simulink model "simulation_from_file"  (Simulink 7.8)
settings: Solver=ode45  StartTime=0.0  StopTime=5.  RelTol=1e-3
settings Model: Creator=roberto  LastModifiedBy=roberto

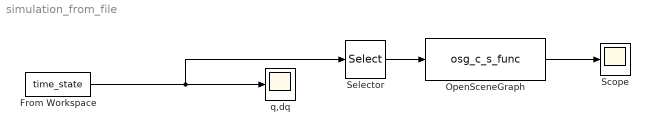
== system simulation_from_file ==
  From Workspace : FromWorkspace  VariableName=time_state  SampleTime=0
  OpenSceneGraph : S-Function  FunctionName=osg_c_s_func  EnableBusSupport=off
  Scope : Scope
  Selector : Selector  InputPortWidth=12  IndexOptions=Index vector (dialog)  Indices=[1 2 3 4 5 6]  OutputSizes=1
  q,dq : Scope
      settings: YMin=-2.5  YMax=2.5  SampleInput=on  SampleTime=0.01
  wires:
  From Workspace/1 -> Selector/1, q,dq/1
  Selector/1 -> OpenSceneGraph/1
  OpenSceneGraph/1 -> Scope/1
